simulink model "SPMSMSensorless"  (R2019b)
settings: Solver=VariableStepAuto  StartTime=0.0  StopTime=10  RelTol=1e-3
undefined symbols (not defined in the file): BmRated, DiscIntNeverNeededParam, etaFSO, etaPsiFSO, JmRated, K_dead, kFSO, KiId, KiIq, KiSpd, KpId, KpIq, kPsiFSO, KpSpd, LdRated, LqRated, OutCur_LowerLimit, OutCur_UpperLimit, OutSpd_LowerLimit, OutSpd_UpperLimit, PhiPMRated, Pn, RsRated, SetSpd_n, TsimCurLoop, TsimMotor, UdcRated, V_dead
libraries: simulink x3, eeTransforms x1, powerlib x1
(part 1 of 2)
settings Model: SimulationMode=accelerator  Creator=Downstream  LastModifiedBy=Downstream
settings DataIOCC: ReturnWorkspaceOutputs=off

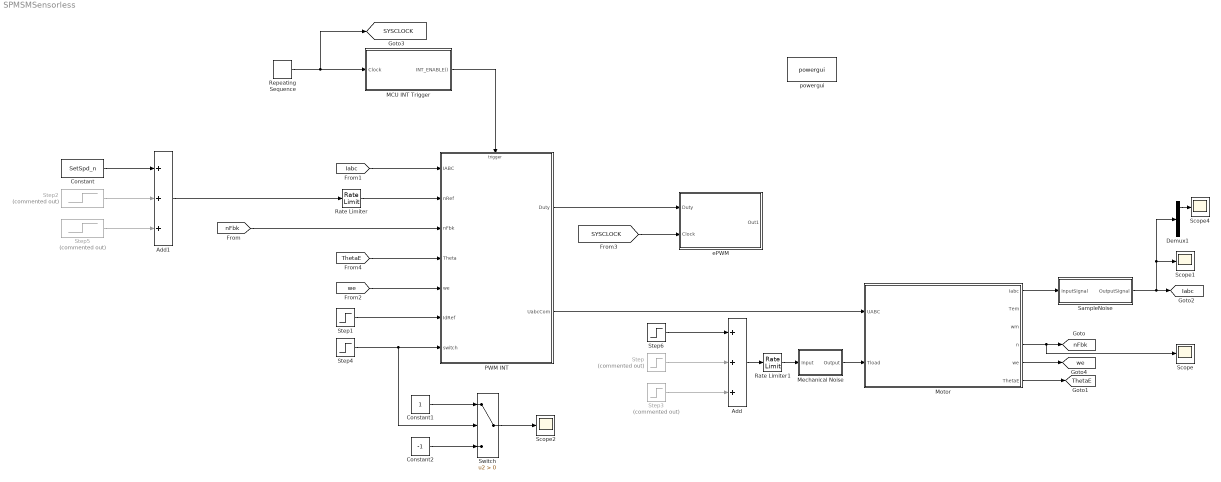
== system SPMSMSensorless ==
  Add : Sum  Inputs=+++
  Add1 : Sum  Inputs=+++
  Constant : Constant  Value=SetSpd_n  SampleTime=-1
  Constant1 : Constant
  Constant2 : Constant  Value=-1
  Demux1 : Demux  Outputs=3
  MCU INT Trigger : MATLAB Function  TreatAsAtomicUnit=on
  Mechanical Noise : Subsystem
  Motor : Subsystem
  PWM INT : Subsystem  TreatAsAtomicUnit=on
  Rate Limiter : RateLimiter  RisingSlewLimit=abs(SetSpd_n)/1  FallingSlewLimit=-abs(SetSpd_n)/1  SampleTimeMode=inherited
  Rate Limiter1 : RateLimiter  RisingSlewLimit=3  FallingSlewLimit=-3  SampleTimeMode=inherited
  Repeating Sequence : simulink/Sources/Repeating Sequence  rep_seq_t=[0 0.5*TsimCurLoop 1*TsimCurLoop]  rep_seq_y=[0 1 0]
  SampleNoise : Subsystem
  Scope{,1..2,4} (4 alike) : Scope
  Step : Step  Commented=on  Time=4  After=1.5  SampleTime=0
  Step1 : Step  Time=5  After=0  SampleTime=0
  Step2 : Step  Commented=on  Time=2  After=-SetSpd_n  SampleTime=0
  Step3 : Step  Commented=on  Time=8  After=1.5  SampleTime=0
  Step4 : Step  Time=2  Before=-1
  Step5 : Step  Commented=on  Time=6  After=-SetSpd_n  SampleTime=0
  Step6 : Step  Time=0  After=3  SampleTime=0
  Switch : Switch  Criteria=u2 > Threshold
  ePWM : Subsystem
  powergui : powerlib/powergui  Priority=1  SimulationMode=Continuous  SampleTime=50e-6  frequency=60  Iterations=50  frequencyindice=60  Pbase=100e6  ErrMax=1e-4  UnitsV=kV  UnitsW=MW  buscounter=0  FunctionMessages=off  echomessages=off  EnableUseOfTLC=off  CurrentSourceSwitches=off  DisableSnubberDevices=off  DisableRonSwitches=off  DisableVfSwitches=off  DisplayEquations=off  AutomaticDiscreteSolvers=off  SolverType=Tustin/Backward Euler (TBE)  Interpol=off  ExternalGateDelay=off  methode=off  Ts=100  x0status=blocks  SPID=on  SwTol=0  HookPort=off  NonlinearTolerance=1e-4  nMaxIteration=100  ContinueOnMaxIteration=off  RestoreLinks=warning  ResistiveCurrentMeasurement=off  Frange=[0:2:500]  Ylog=off  Xlog=on  ShowGrid=off  save=off  variable=ZData  structure=Ud_ComP  ZoomFFT=off  StartTime=2  cycles=200  DisplayStyle=3  fundamental=40  FreqAxis=on  MaxFrequency=40*4  frequencyindicesteady=1  RmsSteady=1  display=off
      settings: SourceProductName=Simscape Electrical
  tag scope: Iabc=global, SYSCLOCK=global, ThetaE=global, nFbk=global, we=global
  wires:
  MCU INT Trigger/1(INT_ENABLE()) -> PWM INT/Trigger
  Repeating Sequence/1 -> [SYSCLOCK], MCU INT Trigger/1(Clock)
  Rate Limiter/1 -> PWM INT/2(nRef)
  [ThetaE] -> PWM INT/4(Theta)
  Motor/4(n) -> Scope/1, [nFbk]
  Motor/6(ThetaE) -> [ThetaE]
  Motor/1(Iabc) -> SampleNoise/1(InputSignal)
  SampleNoise/1(OutputSignal) -> Scope1/1, Demux1/1, [Iabc]
  [Iabc] -> PWM INT/1(IABC)
  Motor/5(we) -> [we]
  [we] -> PWM INT/5(we)
  [SYSCLOCK] -> ePWM/2(Clock)
  PWM INT/1(Duty) -> ePWM/1(Duty)
  PWM INT/2(UabcCom) -> Motor/1(UABC)
  Mechanical Noise/1(Output) -> Motor/2(Tload)
  Add/1 -> Rate Limiter1/1
  Demux1/1 -> Scope4/1
  Step6/1 -> Add/1
  Step/1 -> Add/2
  Step1/1 -> PWM INT/6(IdRef)
  Add1/1 -> Rate Limiter/1
  Constant/1 -> Add1/1
  Step2/1 -> Add1/2
  Step4/1 -> Switch/2, PWM INT/7(switch)
  Constant1/1 -> Switch/1
  Constant2/1 -> Switch/3
  Switch/1 -> Scope2/1
  Step3/1 -> Add/3
  [nFbk] -> PWM INT/3(nFbk)
  Step5/1 -> Add1/3
  Rate Limiter1/1 -> Mechanical Noise/1(Input)

== system SPMSMSensorless/Mechanical Noise ==
  Input : Inport
  Add : Sum
  Gain : Gain  Gain=0.25
  Random Number : RandomNumber  Seed=1
  Rate Transition : RateTransition  OutPortSampleTime=TsimSpdLoop
  Output : Outport
  wires:
  Add/1 -> Output/1
  Input/1 -> Add/1
  Random Number/1 -> Gain/1
  Rate Transition/1 -> Add/2
  Gain/1 -> Rate Transition/1

== system SPMSMSensorless/Motor ==
  UABC : Inport
  Tload : Inport  Port=2
  Add : Sum  Inputs=+-
  Clark Transformation : Subsystem
  Demux : Demux  Outputs=3
  Electrical Model : Subsystem
  Inverse Park Transform : eeTransforms/Inverse Park Transform  AxisAlignment=D-axis  PowerInvariant=off
      settings: SourceProductName=Simscape Electrical
  "Mechanical Model " : Subsystem
  Mux : Mux  Inputs=3
  Park Transformation : Subsystem
  Scope{,1..2,4} (4 alike) : Scope
  VSINonlinearity : Subsystem  Commented=on
  Iabc : Outport
  Tem : Outport  Port=2
  wm : Outport  Port=3
  n : Outport  Port=4
  we : Outport  Port=5
  ThetaE : Outport  Port=6
  wires:
  Park Transformation/1(D) -> Scope/1, Electrical Model/1(Ud)
  "Mechanical Model "/4(we) -> Electrical Model/3(we), we/1
  Electrical Model/4(Phiq) -> "Mechanical Model "/4(Phiq)
  Electrical Model/3(Phid) -> "Mechanical Model "/3(Phid)
  Electrical Model/1(Id) -> Mux/1, Scope4/1, "Mechanical Model "/1(id)
  Park Transformation/2(Q) -> Scope2/1, Electrical Model/2(Uq)
  Demux/1 -> Clark Transformation/1(U)
  Electrical Model/2(Iq) -> Scope1/1, Mux/2, "Mechanical Model "/2(iq)
  Clark Transformation/2(Beta) -> Park Transformation/2(Beta)
  "Mechanical Model "/5(ThetaE) -> Inverse Park Transform/2, ThetaE/1, Park Transformation/3(theta)
  "Mechanical Model "/2(wm) -> wm/1
  Add/1 -> Demux/1
  Clark Transformation/1(Alpha) -> Park Transformation/1(Alpha)
  Mux/1 -> Inverse Park Transform/1
  Demux/2 -> Clark Transformation/2(V)
  Demux/3 -> Clark Transformation/3(W)
  VSINonlinearity/1(UError) -> Add/2
  "Mechanical Model "/1(Tem) -> Tem/1
  "Mechanical Model "/3(n) -> n/1
  Tload/1 -> "Mechanical Model "/5(Tload)
  Inverse Park Transform/1 -> VSINonlinearity/1(IABC), Iabc/1
  UABC/1 -> Add/1

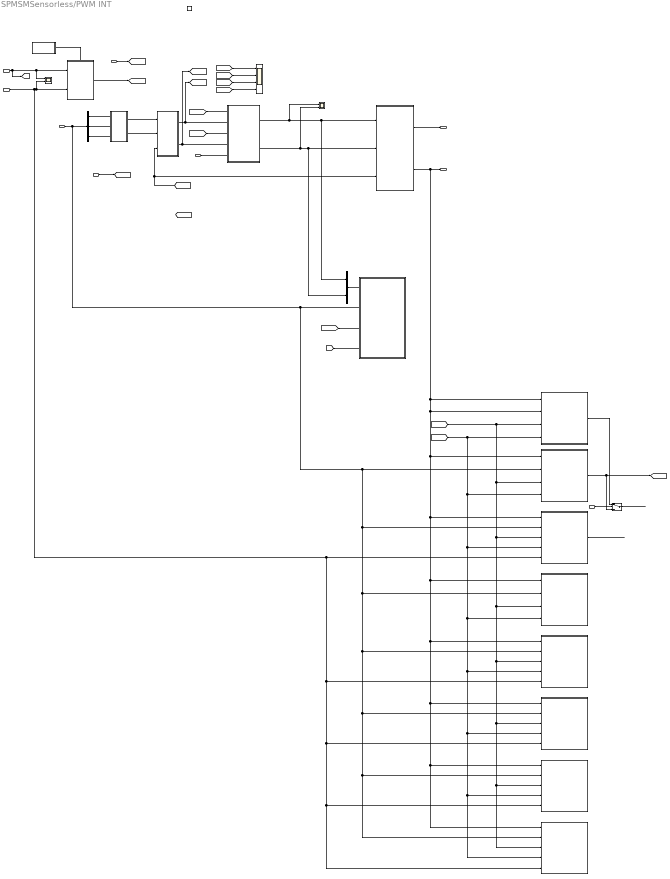
== system SPMSMSensorless/PWM INT ==
  IABC : Inport
  nRef : Inport  Port=2
  nFbk : Inport  Port=3
  Theta : Inport  Port=4
  we : Inport  Port=5
  IdRef : Inport  Port=6
  switch : Inport  Port=7
  function : TriggerPort  TriggerType=function-call  VariantControl=Variant
  Clark Transformation : Subsystem
  CurLoop : Subsystem
  Demux1 : Demux  Outputs=3
  FSO : Subsystem
  FSOLqInf : Subsystem
  FSO_Flux_SpdOb : Subsystem
  FSO_RsInf : Subsystem
  FSO_RsInfPLL : Subsystem
  MATLAB Function : MATLAB Function  TreatAsAtomicUnit=on
  Mux1 : Mux  Inputs=2
  Park Transformation : Subsystem
  PsiFSO : Subsystem
  PsiFSORsAD : Subsystem
  PsiFSORsInf : Subsystem
  "RealVoltageCompesation " : Subsystem  TreatAsAtomicUnit=on
  SVPWM : Subsystem
  Scope : Scope  NumInputPorts=4
  Scope1 : Scope  NumInputPorts=2
  Scope2 : Scope  NumInputPorts=2
  SpdLoop : Subsystem  TreatAsAtomicUnit=on
  Switch : Switch  Criteria=u2 > Threshold
  Duty : Outport
  UabcCom : Outport  Port=2
  wires:
  MATLAB Function/1(SPEED_ENABLE()) -> SpdLoop/Trigger
  nRef/1 -> [nRef], Scope1/1, SpdLoop/1(n_Ref)
  Clark Transformation/2(Beta) -> Park Transformation/2(Beta)
  Clark Transformation/1(Alpha) -> Park Transformation/1(Alpha)
  Demux1/1 -> Clark Transformation/1(U)
  Demux1/2 -> Clark Transformation/2(V)
  Demux1/3 -> Clark Transformation/3(W)
  we/1 -> CurLoop/5(we)
  Park Transformation/1(D) -> [Id_FBK], CurLoop/2(IdFbk)
  Park Transformation/2(Q) -> [Iq_FBK], CurLoop/4(IqFbk)
  SVPWM/1(Duty) -> Duty/1
  [Id_REF] -> CurLoop/1(IdRef)
  [Iq_REF] -> CurLoop/3(IqRef)
  SpdLoop/1(IqRef) -> [Iq_REF]
  IdRef/1 -> [Id_REF]
  [Iq_FBK] -> Scope/2  "IqFbk"
  [Iq_REF] -> Scope/1  "IqRef"
  Mux1/1 -> "RealVoltageCompesation "/1(Udq)
  CurLoop/2(UqCmd) -> Scope2/2, SVPWM/2(Uq), Mux1/2
  CurLoop/1(UdCmd) -> Scope2/1, SVPWM/1(Ud), Mux1/1
  [nRef] -> "RealVoltageCompesation "/4(n)
  [Theta_Est] -> "RealVoltageCompesation "/3(Theta)
  Theta/1 -> [Theta_Real]
  [Theta_Est] -> Park Transformation/3(theta), SVPWM/3(Theta)
  SVPWM/2(UabcCom) -> UabcCom/1, FSOLqInf/1(Uabc), FSOLqInf/2(Iabc), FSO/1(Uabc), PsiFSORsAD/1(Uabc), PsiFSORsInf/1(Uabc), PsiFSO/1(Uabc), FSO_RsInfPLL/1(Uabc), FSO_Flux_SpdOb/1(Uabc), FSO_RsInf/1(Uabc)
  [Id_REF] -> Scope/3  "IdRef"
  [Id_FBK] -> Scope/4  "IdFbk"
  [Theta_Real] -> PsiFSORsAD/4(ThetaReal), PsiFSORsInf/4(ThetaReal), PsiFSO/4(ThetaReal), FSO_RsInfPLL/4(ThetaReal), FSO_Flux_SpdOb/4(ThetaReal), FSO_RsInf/4(ThetaReal), FSO/4(ThetaReal), FSOLqInf/4(ThetaReal)
  [nRef] -> PsiFSO/3(nRef), PsiFSORsInf/3(nRef), PsiFSORsAD/3(nRef), FSO_RsInfPLL/3(nRef), FSO_Flux_SpdOb/3(nRef), FSO_RsInf/3(nRef), FSO/3(nRef), FSOLqInf/3(nRef)
  switch/1 -> Switch/2
  nFbk/1 -> PsiFSORsAD/5("nFbk "), PsiFSORsInf/5("nFbk "), PsiFSO/5("nFbk "), FSO_RsInfPLL/5("nFbk "), FSO_RsInf/5("nFbk "), Scope1/2, SpdLoop/2(n_Fbk)
  IABC/1 -> "RealVoltageCompesation "/2(Iuvw), FSO/2(Iabc), PsiFSORsAD/2(Iabc), PsiFSORsInf/2(Iabc), PsiFSO/2(Iabc), FSO_RsInfPLL/2(Iabc), FSO_Flux_SpdOb/2(Iabc), FSO_RsInf/2(Iabc), Demux1/1
  FSO/1(ThetaEst) -> [Theta_Est], Switch/3
  FSOLqInf/1(ThetaEst) -> Switch/1
  Switch/1 -> ?
  FSO_RsInf/1(ThetaEst) -> ?

== system SPMSMSensorless/SampleNoise ==
  InputSignal : Inport
  Add : Sum
  Add1 : Sum
  Add2 : Sum
  Demux : Demux  Outputs=3
  Gain : Gain  Gain=0.025
  Gain1 : Gain  Gain=0.025
  Gain2 : Gain  Gain=0.025
  Mux : Mux  Inputs=3
  Random Number : RandomNumber  Seed=5
  Random Number1 : RandomNumber  Seed=8
  Random Number2 : RandomNumber  Seed=15
  Scope : Scope
  OutputSignal : Outport
  wires:
  InputSignal/1 -> Demux/1
  Random Number/1 -> Gain/1
  Random Number1/1 -> Gain1/1
  Random Number2/1 -> Gain2/1
  Demux/1 -> Add/1
  Gain/1 -> Scope/1, Add/2
  Demux/2 -> Add1/1
  Demux/3 -> Add2/1
  Gain1/1 -> Add1/2
  Gain2/1 -> Add2/2
  Add/1 -> Mux/1
  Add1/1 -> Mux/2
  Add2/1 -> Mux/3
  Mux/1 -> OutputSignal/1

== system SPMSMSensorless/ePWM ==
  Duty : Inport
  Clock : Inport  Port=2
  Add : Sum  Inputs=+-
  Add1 : Sum  Inputs=+-
  Add2 : Sum  Inputs=+-
  Demux : Demux  Outputs=3
  Gain : Gain  Gain=UdcRated/2
  Mux : Mux  Inputs=3
  Relay : Relay  OnSwitchValue=0  OffSwitchValue=0  OffOutputValue=-1
  Relay1 : Relay  OnSwitchValue=0  OffSwitchValue=0  OffOutputValue=-1
  Relay2 : Relay  OnSwitchValue=0  OffSwitchValue=0  OffOutputValue=-1
  Out1 : Outport
  wires:
  Duty/1 -> Demux/1
  Demux/1 -> Add/1
  Demux/2 -> Add1/1
  Demux/3 -> Add2/1
  Clock/1 -> Add/2, Add1/2, Add2/2
  Add/1 -> Relay/1
  Add1/1 -> Relay1/1
  Add2/1 -> Relay2/1
  Relay/1 -> Mux/1
  Relay1/1 -> Mux/2
  Relay2/1 -> Mux/3
  Mux/1 -> Gain/1
  Gain/1 -> Out1/1

== system SPMSMSensorless/Motor/Clark Transformation ==
  U : Inport
  V : Inport  Port=2
  W : Inport  Port=3
  Add : Sum  Inputs=+--
  Add1 : Sum  Inputs=+-
  Gain : Gain  Gain=0.5
  Gain1 : Gain  Gain=0.5
  Gain2 : Gain  Gain=2/3
  Gain3 : Gain  Gain=2/3*0.86602540
  Alpha : Outport
  Beta : Outport  Port=2
  wires:
  V/1 -> Add1/1, Gain/1
  Gain/1 -> Add/2
  W/1 -> Add1/2, Gain1/1
  Gain1/1 -> Add/3
  U/1 -> Add/1
  Add/1 -> Gain2/1
  Gain2/1 -> Alpha/1
  Add1/1 -> Gain3/1
  Gain3/1 -> Beta/1

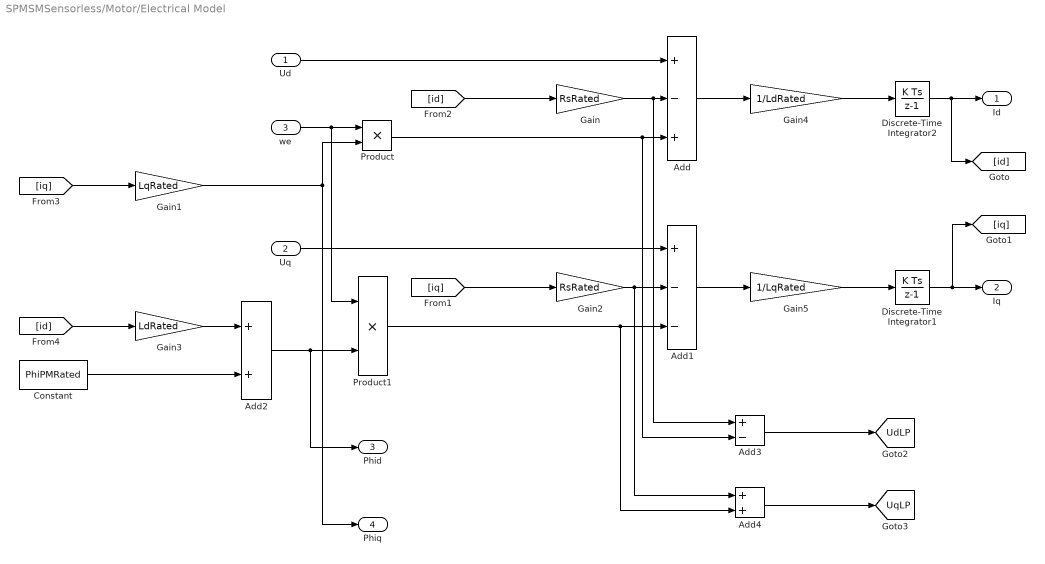
== system SPMSMSensorless/Motor/Electrical Model ==
  Ud : Inport
  Uq : Inport  Port=2
  we : Inport  Port=3
  Add : Sum  Inputs=+-+
  Add1 : Sum  Inputs=+--
  Add2 : Sum
  Add3 : Sum  Inputs=+-
  Add4 : Sum
  Constant : Constant  Value=PhiPMRated  SampleTime=TsimMotor
  Discrete-Time Integrator1 : DiscreteIntegrator  InitialCondition=1  SampleTime=TsimMotor  UpperSaturationLimit=0  LowerSaturationLimit=-400  ICPrevOutput=DiscIntNeverNeededParam  ICPrevScaledInput=DiscIntNeverNeededParam
  Discrete-Time Integrator2 : DiscreteIntegrator  InitialCondition=1  SampleTime=TsimMotor  UpperSaturationLimit=0  LowerSaturationLimit=-400  ICPrevOutput=DiscIntNeverNeededParam  ICPrevScaledInput=DiscIntNeverNeededParam
  Gain : Gain  Gain=RsRated
  Gain1 : Gain  Gain=LqRated
  Gain2 : Gain  Gain=RsRated
  Gain3 : Gain  Gain=LdRated
  Gain4 : Gain  Gain=1/LdRated
  Gain5 : Gain  Gain=1/LqRated
  Product : Product
  Product1 : Product
  Id : Outport
  Iq : Outport  Port=2
  Phid : Outport  Port=3
  Phiq : Outport  Port=4
  tag scope: UdLP=global, UqLP=global
  wires:
  Ud/1 -> Add/1
  we/1 -> Product/1, Product1/1
  Gain/1 -> Add3/1, Add/2
  [iq] -> Gain1/1
  [id] -> Gain/1
  Add/1 -> Gain4/1
  [id] -> Gain3/1
  [iq] -> Gain2/1
  Gain2/1 -> Add4/1, Add1/2
  Uq/1 -> Add1/1
  Gain3/1 -> Add2/1
  Constant/1 -> Add2/2
  Add2/1 -> Phid/1, Product1/2
  Product1/1 -> Add4/2, Add1/3
  Add1/1 -> Gain5/1
  Gain4/1 -> Discrete-Time Integrator2/1
  Gain5/1 -> Discrete-Time Integrator1/1
  Discrete-Time Integrator2/1 -> [id], Id/1
  Discrete-Time Integrator1/1 -> [iq], Iq/1
  Gain1/1 -> Phiq/1, Product/2
  Product/1 -> Add/3, Add3/2
  Add3/1 -> [UdLP]
  Add4/1 -> [UqLP]

== system SPMSMSensorless/Motor/Mechanical Model  ==
  id : Inport
  iq : Inport  Port=2
  Phid : Inport  Port=3
  Phiq : Inport  Port=4
  Tload : Inport  Port=5
  Add : Sum  Inputs=+-
  Add1 : Sum  Inputs=+--
  Discrete-Time Integrator1 : DiscreteIntegrator  SampleTime=TsimMotor  ICPrevOutput=DiscIntNeverNeededParam  ICPrevScaledInput=DiscIntNeverNeededParam
  Discrete-Time Integrator2 : DiscreteIntegrator  InitialCondition=SetSpd_n/60*2*pi  SampleTime=TsimMotor  ICPrevOutput=DiscIntNeverNeededParam  ICPrevScaledInput=DiscIntNeverNeededParam
  Gain : Gain  Gain=1.5*Pn
  Gain1 : Gain  Gain=60/2/pi
  Gain2 : Gain  Gain=Pn
  Gain3 : Gain  Gain=1/JmRated
  Gain4 : Gain  Gain=BmRated
  Product : Product
  Product1 : Product
  Tem : Outport
  wm : Outport  Port=2
  n : Outport  Port=3
  we : Outport  Port=4
  ThetaE : Outport  Port=5
  wires:
  iq/1 -> Product/1
  Phid/1 -> Product/2
  Phiq/1 -> Product1/2
  id/1 -> Product1/1
  Product/1 -> Add/1
  Product1/1 -> Add/2
  Add/1 -> Gain/1
  Gain/1 -> Tem/1, Add1/1
  Tload/1 -> Add1/2
  Add1/1 -> Gain3/1
  Gain3/1 -> Discrete-Time Integrator2/1
  Gain1/1 -> n/1
  Gain2/1 -> Discrete-Time Integrator1/1, we/1
  Discrete-Time Integrator1/1 -> ThetaE/1
  Gain4/1 -> Add1/3
  Discrete-Time Integrator2/1 -> wm/1, Gain4/1, Gain2/1, Gain1/1

== system SPMSMSensorless/Motor/Park Transformation ==
  Alpha : Inport
  Beta : Inport  Port=2
  theta : Inport  Port=3
  Add : Sum
  Add1 : Sum  Inputs=+-
  Product{,1..3} (4 alike) : Product
  Sin : Trigonometry  OutputSignalType=real
  Sin1 : Trigonometry  Operator=cos  OutputSignalType=real
  D : Outport
  Q : Outport  Port=2
  wires:
  Product/1 -> Add/1
  Sin/1 -> Product3/2, Product1/2
  Product1/1 -> Add/2
  Add1/1 -> Q/1
  Sin1/1 -> Product2/2, Product/2
  Product2/1 -> Add1/1
  Alpha/1 -> Product3/1, Product/1
  Beta/1 -> Product2/1, Product1/1
  Product3/1 -> Add1/2
  Add/1 -> D/1
  theta/1 -> Sin/1, Sin1/1

== system SPMSMSensorless/Motor/VSINonlinearity ==
  IABC : Inport
  Constant : Constant  Value=K_dead  SampleTime=TsimMotor
  Constant1 : Constant  Value=V_dead  SampleTime=TsimMotor
  Demux1 : Demux  Outputs=3
  MATLAB Function1 : MATLAB Function  TreatAsAtomicUnit=on
  MATLAB Function2 : MATLAB Function  TreatAsAtomicUnit=on
  MATLAB Function3 : MATLAB Function  TreatAsAtomicUnit=on
  Mux1 : Mux  Inputs=3
  Scope : Scope
  UError : Outport
  wires:
  Demux1/3 -> MATLAB Function3/1(I)
  Constant1/1 -> MATLAB Function3/3(Vdead), MATLAB Function2/3(Vdead), MATLAB Function1/3(Vdead)
  Constant/1 -> MATLAB Function3/2(K), MATLAB Function2/2(K), MATLAB Function1/2(K)
  MATLAB Function3/1(U) -> Mux1/3
  Demux1/2 -> MATLAB Function2/1(I)
  MATLAB Function2/1(U) -> Mux1/2
  Demux1/1 -> MATLAB Function1/1(I)
  Mux1/1 -> UError/1
  IABC/1 -> Demux1/1
  MATLAB Function1/1(U) -> Scope/1, Mux1/1

== system SPMSMSensorless/PWM INT/Clark Transformation ==
  U : Inport
  V : Inport  Port=2
  W : Inport  Port=3
  Add : Sum  Inputs=+--
  Add1 : Sum  Inputs=+-
  Gain : Gain  Gain=0.5
  Gain1 : Gain  Gain=0.5
  Gain2 : Gain  Gain=2/3
  Gain3 : Gain  Gain=2/3*0.86602540
  Alpha : Outport
  Beta : Outport  Port=2
  wires:
  V/1 -> Add1/1, Gain/1
  Gain/1 -> Add/2
  W/1 -> Add1/2, Gain1/1
  Gain1/1 -> Add/3
  U/1 -> Add/1
  Add/1 -> Gain2/1
  Gain2/1 -> Alpha/1
  Add1/1 -> Gain3/1
  Gain3/1 -> Beta/1

== system SPMSMSensorless/PWM INT/CurLoop ==
  IdRef : Inport
  IdFbk : Inport  Port=2
  IqRef : Inport  Port=3
  IqFbk : Inport  Port=4
  we : Inport  Port=5
  Add : Sum
  Constant2 : Constant  Value=PhiPMRated  SampleTime=-1
  Gain : Gain  Gain=LqRated
  Gain2 : Gain  Gain=-1
  Gain3 : Gain  Gain=LdRated
  PI_Id : Subsystem
  PI_Iq : Subsystem
  Product : Product
  Product3 : Product
  Saturation : Saturate  UpperLimit=OutCur_UpperLimit  LowerLimit=OutCur_LowerLimit
  Saturation1 : Saturate  UpperLimit=OutCur_UpperLimit  LowerLimit=OutCur_LowerLimit
  Sum : Sum  Inputs=|++
  Sum1 : Sum  Inputs=++|
  UdCmd : Outport
  UqCmd : Outport  Port=2
  wires:
  Gain/1 -> Product/1
  IdFbk/1 -> Gain3/1, PI_Id/2("Id_Fbk ")
  Sum/1 -> Saturation1/1
  PI_Id/1(PI_IdOut) -> Sum/1
  Product/1 -> Gain2/1
  IdRef/1 -> PI_Id/1(Id_Ref)
  Gain2/1 -> Sum/2
  Sum1/1 -> Saturation/1
  Saturation1/1 -> UdCmd/1
  Saturation/1 -> UqCmd/1
  IqRef/1 -> PI_Iq/1(Iq_Ref)
  PI_Iq/1(PI_IqOut) -> Sum1/2
  IqFbk/1 -> Gain/1, PI_Iq/2("Iq_Fbk ")
  Add/1 -> Product3/2
  Gain3/1 -> Add/1
  Constant2/1 -> Add/2
  Product3/1 -> Sum1/1
  we/1 -> Product3/1, Product/2

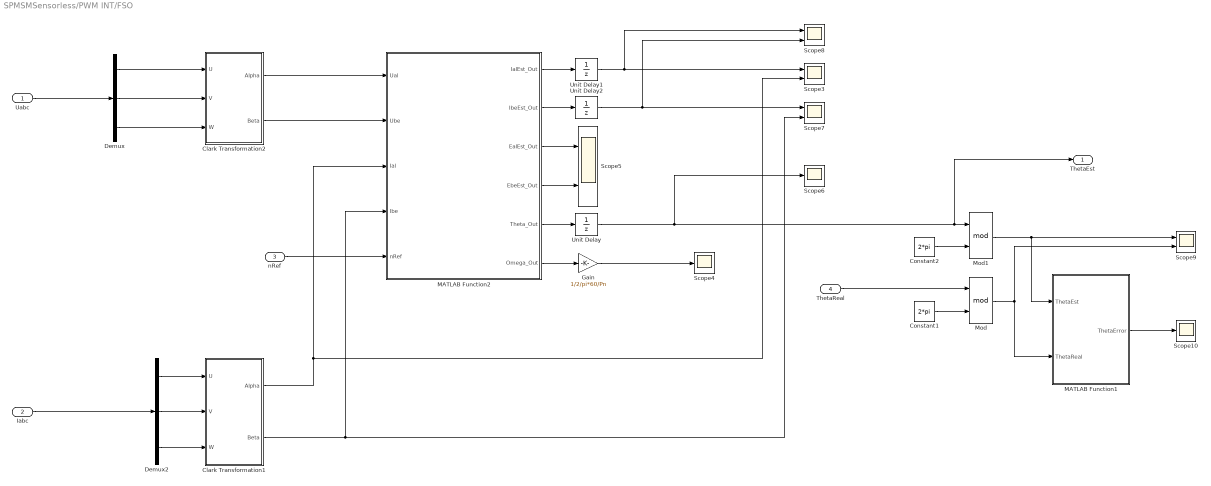
== system SPMSMSensorless/PWM INT/FSO ==
  Uabc : Inport
  Iabc : Inport  Port=2
  nRef : Inport  Port=3
  ThetaReal : Inport  Port=4
  Clark Transformation1 : Subsystem
  Clark Transformation2 : Subsystem
  Constant1 : Constant  Value=2*pi  SampleTime=-1
  Constant2 : Constant  Value=2*pi  SampleTime=-1
  Demux : Demux  Outputs=3
  Demux2 : Demux  Outputs=3
  Gain : Gain  Gain=1/2/pi*60/Pn
  MATLAB Function1 : MATLAB Function  TreatAsAtomicUnit=on
  MATLAB Function2 : MATLAB Function  TreatAsAtomicUnit=on
  Mod : Math  Operator=mod  SignedPower=off  SaturateOnIntegerOverflow=on
  Mod1 : Math  Operator=mod  SignedPower=off  SaturateOnIntegerOverflow=on
  Scope10 : Scope
  Scope{3,5,7..9} (5 alike) : Scope  NumInputPorts=2
  Scope4 : Scope
  Scope6 : Scope
  Unit Delay : UnitDelay  SampleTime=-1  HasFrameUpgradeWarning=on
  Unit Delay1 : UnitDelay  SampleTime=-1  HasFrameUpgradeWarning=on
  Unit Delay2 : UnitDelay  SampleTime=-1  HasFrameUpgradeWarning=on
  ThetaEst : Outport
  wires:
  Constant1/1 -> Mod/2
  MATLAB Function2/6(Omega_Out) -> Gain/1
  Demux2/2 -> Clark Transformation1/2(V)
  Mod1/1 -> MATLAB Function1/1(ThetaEst), Scope9/1
  Unit Delay2/1 -> Scope8/2, Scope7/1
  Clark Transformation2/2(Beta) -> MATLAB Function2/2(Ube)
  Demux2/1 -> Clark Transformation1/1(U)
  Clark Transformation1/2(Beta) -> MATLAB Function2/4(Ibe), Scope7/2
  Uabc/1 -> Demux/1
  MATLAB Function2/2(IbeEst_Out) -> Unit Delay2/1
  Iabc/1 -> Demux2/1
  MATLAB Function2/3(EalEst_Out) -> Scope5/1
  Mod/1 -> MATLAB Function1/2(ThetaReal), Scope9/2
  Demux2/3 -> Clark Transformation1/3(W)
  Demux/3 -> Clark Transformation2/3(W)
  Gain/1 -> Scope4/1
  Unit Delay1/1 -> Scope8/1, Scope3/1
  MATLAB Function2/1(IalEst_Out) -> Unit Delay1/1
  MATLAB Function1/1(ThetaError) -> Scope10/1
  Clark Transformation1/1(Alpha) -> MATLAB Function2/3(Ial), Scope3/2
  Demux/1 -> Clark Transformation2/1(U)
  MATLAB Function2/5(Theta_Out) -> Unit Delay/1
  Unit Delay/1 -> Scope6/1, ThetaEst/1, Mod1/1
  Constant2/1 -> Mod1/2
  MATLAB Function2/4(EbeEst_Out) -> Scope5/2
  Demux/2 -> Clark Transformation2/2(V)
  ThetaReal/1 -> Mod/1
  nRef/1 -> MATLAB Function2/5(nRef)
  Clark Transformation2/1(Alpha) -> MATLAB Function2/1(Ual)

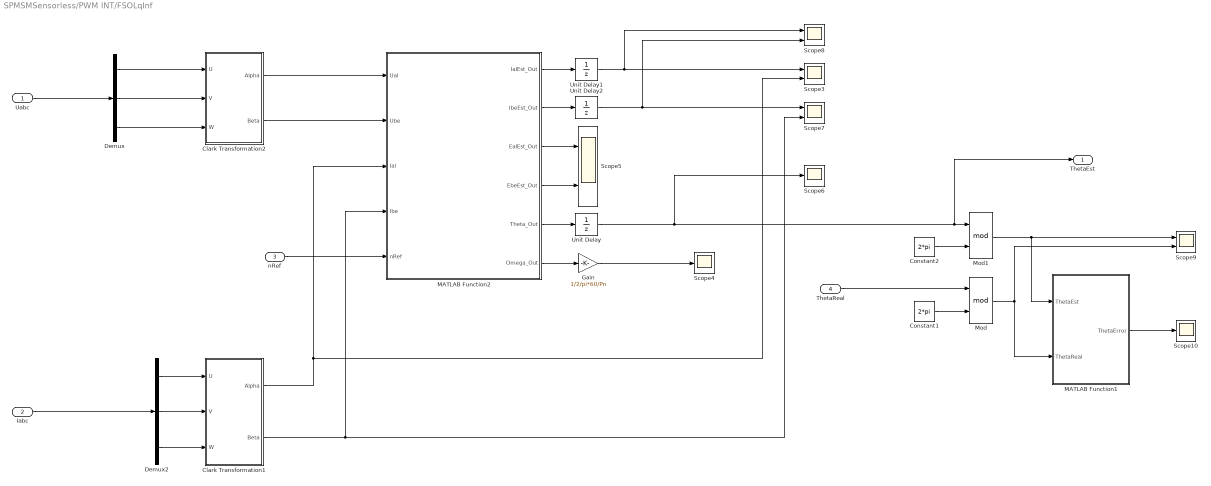
== system SPMSMSensorless/PWM INT/FSOLqInf ==
  Uabc : Inport
  Iabc : Inport  Port=2
  nRef : Inport  Port=3
  ThetaReal : Inport  Port=4
  Clark Transformation1 : Subsystem
  Clark Transformation2 : Subsystem
  Constant1 : Constant  Value=2*pi  SampleTime=-1
  Constant2 : Constant  Value=2*pi  SampleTime=-1
  Demux : Demux  Outputs=3
  Demux2 : Demux  Outputs=3
  Gain : Gain  Gain=1/2/pi*60/Pn
  MATLAB Function1 : MATLAB Function  TreatAsAtomicUnit=on
  MATLAB Function2 : MATLAB Function  TreatAsAtomicUnit=on
  Mod : Math  Operator=mod  SignedPower=off  SaturateOnIntegerOverflow=on
  Mod1 : Math  Operator=mod  SignedPower=off  SaturateOnIntegerOverflow=on
  Scope10 : Scope
  Scope{3,5,7..9} (5 alike) : Scope  NumInputPorts=2
  Scope4 : Scope
  Scope6 : Scope
  Unit Delay : UnitDelay  SampleTime=-1  HasFrameUpgradeWarning=on
  Unit Delay1 : UnitDelay  SampleTime=-1  HasFrameUpgradeWarning=on
  Unit Delay2 : UnitDelay  SampleTime=-1  HasFrameUpgradeWarning=on
  ThetaEst : Outport
  wires:
  Clark Transformation2/1(Alpha) -> MATLAB Function2/1(Ual)
  nRef/1 -> MATLAB Function2/5(nRef)
  ThetaReal/1 -> Mod/1
  Demux/2 -> Clark Transformation2/2(V)
  MATLAB Function2/4(EbeEst_Out) -> Scope5/2
  Constant2/1 -> Mod1/2
  Unit Delay/1 -> Mod1/1, ThetaEst/1, Scope6/1
  MATLAB Function2/5(Theta_Out) -> Unit Delay/1
  Demux/1 -> Clark Transformation2/1(U)
  Clark Transformation1/1(Alpha) -> Scope3/2, MATLAB Function2/3(Ial)
  MATLAB Function1/1(ThetaError) -> Scope10/1
  MATLAB Function2/1(IalEst_Out) -> Unit Delay1/1
  Unit Delay1/1 -> Scope3/1, Scope8/1
  Gain/1 -> Scope4/1
  Demux/3 -> Clark Transformation2/3(W)
  Demux2/3 -> Clark Transformation1/3(W)
  Mod/1 -> Scope9/2, MATLAB Function1/2(ThetaReal)
  MATLAB Function2/3(EalEst_Out) -> Scope5/1
  Iabc/1 -> Demux2/1
  MATLAB Function2/2(IbeEst_Out) -> Unit Delay2/1
  Uabc/1 -> Demux/1
  Clark Transformation1/2(Beta) -> Scope7/2, MATLAB Function2/4(Ibe)
  Demux2/1 -> Clark Transformation1/1(U)
  Clark Transformation2/2(Beta) -> MATLAB Function2/2(Ube)
  Unit Delay2/1 -> Scope7/1, Scope8/2
  Mod1/1 -> Scope9/1, MATLAB Function1/1(ThetaEst)
  Demux2/2 -> Clark Transformation1/2(V)
  MATLAB Function2/6(Omega_Out) -> Gain/1
  Constant1/1 -> Mod/2

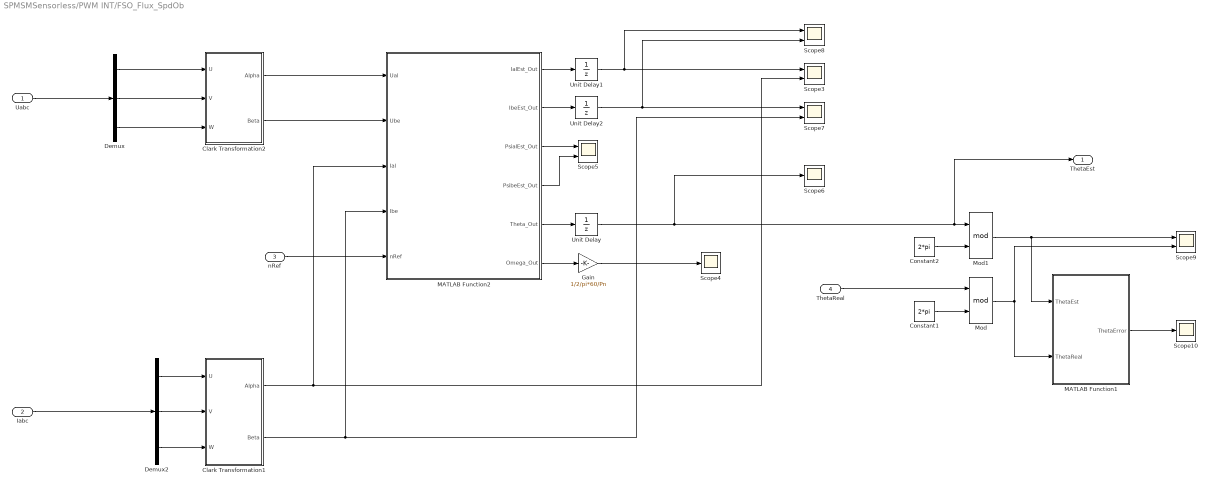
== system SPMSMSensorless/PWM INT/FSO_Flux_SpdOb ==
  Uabc : Inport
  Iabc : Inport  Port=2
  nRef : Inport  Port=3
  ThetaReal : Inport  Port=4
  Clark Transformation1 : Subsystem
  Clark Transformation2 : Subsystem
  Constant1 : Constant  Value=2*pi  SampleTime=-1
  Constant2 : Constant  Value=2*pi  SampleTime=-1
  Demux : Demux  Outputs=3
  Demux2 : Demux  Outputs=3
  Gain : Gain  Gain=1/2/pi*60/Pn
  MATLAB Function1 : MATLAB Function  TreatAsAtomicUnit=on
  MATLAB Function2 : MATLAB Function  TreatAsAtomicUnit=on
  Mod : Math  Operator=mod  SignedPower=off  SaturateOnIntegerOverflow=on
  Mod1 : Math  Operator=mod  SignedPower=off  SaturateOnIntegerOverflow=on
  Scope10 : Scope
  Scope{3,5,7..9} (5 alike) : Scope  NumInputPorts=2
  Scope4 : Scope
  Scope6 : Scope
  Unit Delay : UnitDelay  SampleTime=-1  HasFrameUpgradeWarning=on
  Unit Delay1 : UnitDelay  SampleTime=-1  HasFrameUpgradeWarning=on
  Unit Delay2 : UnitDelay  SampleTime=-1  HasFrameUpgradeWarning=on
  ThetaEst : Outport
  wires:
  Clark Transformation2/1(Alpha) -> MATLAB Function2/1(Ual)
  nRef/1 -> MATLAB Function2/5(nRef)
  ThetaReal/1 -> Mod/1
  Demux/2 -> Clark Transformation2/2(V)
  MATLAB Function2/4(PsibeEst_Out) -> Scope5/2
  Constant2/1 -> Mod1/2
  Unit Delay/1 -> Mod1/1, ThetaEst/1, Scope6/1
  MATLAB Function2/5(Theta_Out) -> Unit Delay/1
  Demux/1 -> Clark Transformation2/1(U)
  Clark Transformation1/1(Alpha) -> Scope3/2, MATLAB Function2/3(Ial)
  MATLAB Function1/1(ThetaError) -> Scope10/1
  MATLAB Function2/1(IalEst_Out) -> Unit Delay1/1
  Unit Delay1/1 -> Scope3/1, Scope8/1
  Gain/1 -> Scope4/1
  Demux/3 -> Clark Transformation2/3(W)
  Demux2/3 -> Clark Transformation1/3(W)
  Mod/1 -> Scope9/2, MATLAB Function1/2(ThetaReal)
  MATLAB Function2/3(PsialEst_Out) -> Scope5/1
  Iabc/1 -> Demux2/1
  MATLAB Function2/2(IbeEst_Out) -> Unit Delay2/1
  Uabc/1 -> Demux/1
  Clark Transformation1/2(Beta) -> Scope7/2, MATLAB Function2/4(Ibe)
  Demux2/1 -> Clark Transformation1/1(U)
  Clark Transformation2/2(Beta) -> MATLAB Function2/2(Ube)
  Unit Delay2/1 -> Scope7/1, Scope8/2
  Mod1/1 -> Scope9/1, MATLAB Function1/1(ThetaEst)
  Demux2/2 -> Clark Transformation1/2(V)
  MATLAB Function2/6(Omega_Out) -> Gain/1
  Constant1/1 -> Mod/2

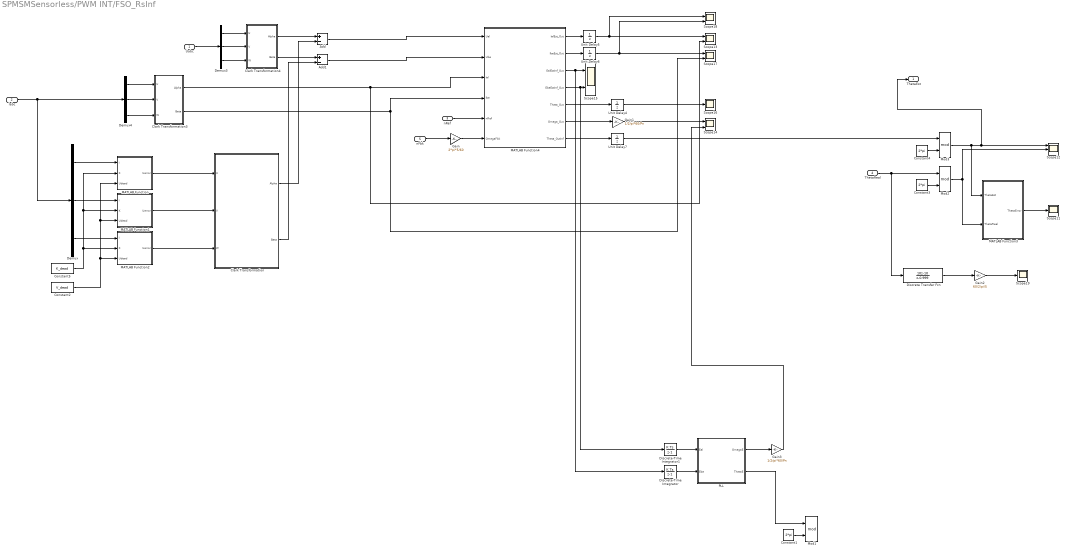
== system SPMSMSensorless/PWM INT/FSO_RsInf ==
  Uabc : Inport
  Iabc : Inport  Port=2
  nRef : Inport  Port=3
  ThetaReal : Inport  Port=4
  "nFbk " : Inport  Port=5
  Add : Sum  Inputs=+-
  Add1 : Sum  Inputs=+-
  Clark Transformation : Subsystem
  Clark Transformation3 : Subsystem
  Clark Transformation4 : Subsystem
  Constant1 : Constant  Value=2*pi  SampleTime=-1
  Constant2 : Constant  Value=V_dead  SampleTime=-1
  Constant3 : Constant  Value=2*pi  SampleTime=-1
  Constant4 : Constant  Value=2*pi  SampleTime=-1
  Constant5 : Constant  Value=K_dead  SampleTime=-1
  Demux : Demux  Outputs=3
  Demux3 : Demux  Outputs=3
  Demux4 : Demux  Outputs=3
  Discrete Transfer Fcn : DiscreteTransferFcn  Numerator=[10 -10]  Denominator=[1 -0.999]
  Discrete-Time Integrator : DiscreteIntegrator  SampleTime=-1  ICPrevOutput=DiscIntNeverNeededParam  ICPrevScaledInput=DiscIntNeverNeededParam
  Discrete-Time Integrator1 : DiscreteIntegrator  SampleTime=-1  ICPrevOutput=DiscIntNeverNeededParam  ICPrevScaledInput=DiscIntNeverNeededParam
  Gain : Gain  Gain=2*pi*5/60
  Gain1 : Gain  Gain=1/2/pi*60/Pn
  Gain2 : Gain  Gain=60/2/pi/5
  Gain3 : Gain  Gain=1/2/pi*60/Pn
  MATLAB Function : MATLAB Function  TreatAsAtomicUnit=on
  MATLAB Function1 : MATLAB Function  TreatAsAtomicUnit=on
  MATLAB Function2 : MATLAB Function  TreatAsAtomicUnit=on
  MATLAB Function3 : MATLAB Function  TreatAsAtomicUnit=on
  MATLAB Function4 : MATLAB Function  TreatAsAtomicUnit=on
  Mod1 : Math  Operator=mod  SignedPower=off  SaturateOnIntegerOverflow=on
  Mod2 : Math  Operator=mod  SignedPower=off  SaturateOnIntegerOverflow=on
  Mod3 : Math  Operator=mod  SignedPower=off  SaturateOnIntegerOverflow=on
  PLL : Subsystem
  Scope11 : Scope
  Scope12 : Scope  NumInputPorts=3
  Scope{13..15,17..18} (5 alike) : Scope  NumInputPorts=2
  Scope16 : Scope
  Scope19 : Scope
  Unit Delay{4..7} (4 alike) : UnitDelay  SampleTime=-1  HasFrameUpgradeWarning=on
  ThetaEst : Outport
  wires:
  ThetaReal/1 -> Discrete Transfer Fcn/1, Mod2/1
  Mod2/1 -> MATLAB Function3/2(ThetaReal), Scope12/2
  Demux3/2 -> Clark Transformation4/2(V)
  Constant3/1 -> Mod2/2
  Gain2/1 -> Scope19/1
  Unit Delay7/1 -> Mod3/1
  Uabc/1 -> Demux3/1
  Mod3/1 -> MATLAB Function3/1(ThetaEst), ThetaEst/1, Scope12/1
  MATLAB Function4/5(Theta_Out) -> Unit Delay4/1
  Clark Transformation3/1(Alpha) -> MATLAB Function4/3(Ial), Scope13/2
  Constant4/1 -> Mod3/2
  Unit Delay6/1 -> Scope18/2, Scope17/1
  Demux4/2 -> Clark Transformation3/2(V)
  Demux3/3 -> Clark Transformation4/3(W)
  MATLAB Function4/1(IalEst_Out) -> Unit Delay5/1
  Unit Delay4/1 -> Scope16/1
  Discrete Transfer Fcn/1 -> Gain2/1
  MATLAB Function3/1(ThetaError) -> Scope11/1
  Demux4/1 -> Clark Transformation3/1(U)
  MATLAB Function4/4(EbeEstInf_Out) -> Discrete-Time Integrator1/1, Scope15/2
  MATLAB Function4/6(Omega_Out) -> Gain1/1
  Demux3/1 -> Clark Transformation4/1(U)
  MATLAB Function4/7(Theta_OutInf) -> Unit Delay7/1
  MATLAB Function4/3(EalEstInf_Out) -> Discrete-Time Integrator/1, Scope15/1
  Demux4/3 -> Clark Transformation3/3(W)
  MATLAB Function4/2(IbeEst_Out) -> Unit Delay6/1
  Clark Transformation3/2(Beta) -> MATLAB Function4/4(Ibe), Scope17/2
  Unit Delay5/1 -> Scope13/1, Scope18/1
  Gain1/1 -> Scope14/1
  nRef/1 -> MATLAB Function4/5(nRef)
  "nFbk "/1 -> Gain/1
  Gain/1 -> MATLAB Function4/6(OmegaFbk)
  PLL/1(OmegaE) -> Gain3/1
  Gain3/1 -> Scope14/2
  Constant1/1 -> Mod1/2
  PLL/2(ThetaE) -> Mod1/1
  Discrete-Time Integrator/1 -> PLL/2(Ebe)
  Discrete-Time Integrator1/1 -> PLL/1(Eal)
  Constant2/1 -> MATLAB Function2/3(Udead), MATLAB Function1/3(Udead), MATLAB Function/3(Udead)
  Constant5/1 -> MATLAB Function2/2(K), MATLAB Function1/2(K), MATLAB Function/2(K)
  MATLAB Function2/1(Uerror) -> Clark Transformation/3(W)
  Demux/2 -> MATLAB Function1/1(I)
  Demux/1 -> MATLAB Function/1(I)
  MATLAB Function/1(Uerror) -> Clark Transformation/1(U)
  Iabc/1 -> Demux/1, Demux4/1
  MATLAB Function1/1(Uerror) -> Clark Transformation/2(V)
  Demux/3 -> MATLAB Function2/1(I)
  Clark Transformation/1(Alpha) -> Add/2
  Clark Transformation4/1(Alpha) -> Add/1
  Add/1 -> MATLAB Function4/1(Ual)
  Clark Transformation4/2(Beta) -> Add1/1
  Add1/1 -> MATLAB Function4/2(Ube)
  Clark Transformation/2(Beta) -> Add1/2

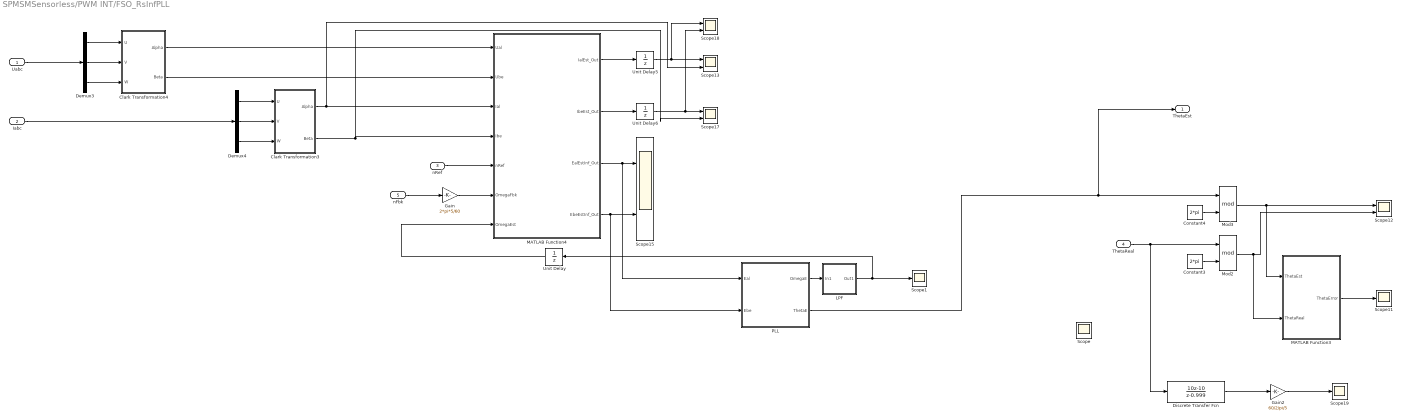
== system SPMSMSensorless/PWM INT/FSO_RsInfPLL ==
  Uabc : Inport
  Iabc : Inport  Port=2
  nRef : Inport  Port=3
  ThetaReal : Inport  Port=4
  "nFbk " : Inport  Port=5
  Clark Transformation3 : Subsystem
  Clark Transformation4 : Subsystem
  Constant3 : Constant  Value=2*pi  SampleTime=-1
  Constant4 : Constant  Value=2*pi  SampleTime=-1
  Demux3 : Demux  Outputs=3
  Demux4 : Demux  Outputs=3
  Discrete Transfer Fcn : DiscreteTransferFcn  Numerator=[10 -10]  Denominator=[1 -0.999]
  Gain : Gain  Gain=2*pi*5/60
  Gain2 : Gain  Gain=60/2/pi/5
  LPF : Subsystem
  MATLAB Function3 : MATLAB Function  TreatAsAtomicUnit=on
  MATLAB Function4 : MATLAB Function  TreatAsAtomicUnit=on
  Mod2 : Math  Operator=mod  SignedPower=off  SaturateOnIntegerOverflow=on
  Mod3 : Math  Operator=mod  SignedPower=off  SaturateOnIntegerOverflow=on
  PLL : Subsystem
  Scope{,1,11,19} (4 alike) : Scope
  Scope{12..13,15,17..18} (5 alike) : Scope  NumInputPorts=2
  Unit Delay : UnitDelay  SampleTime=-1  HasFrameUpgradeWarning=on
  Unit Delay5 : UnitDelay  SampleTime=-1  HasFrameUpgradeWarning=on
  Unit Delay6 : UnitDelay  SampleTime=-1  HasFrameUpgradeWarning=on
  ThetaEst : Outport
  wires:
  Gain/1 -> MATLAB Function4/6(OmegaFbk)
  "nFbk "/1 -> Gain/1
  Unit Delay5/1 -> Scope18/1, Scope13/1
  Clark Transformation3/2(Beta) -> Scope17/2, MATLAB Function4/4(Ibe)
  MATLAB Function4/2(IbeEst_Out) -> Unit Delay6/1
  Demux4/3 -> Clark Transformation3/3(W)
  MATLAB Function4/3(EalEstInf_Out) -> PLL/1(Eal), Scope15/1
  Demux3/1 -> Clark Transformation4/1(U)
  MATLAB Function4/4(EbeEstInf_Out) -> PLL/2(Ebe), Scope15/2
  Demux4/1 -> Clark Transformation3/1(U)
  MATLAB Function3/1(ThetaError) -> Scope11/1
  Discrete Transfer Fcn/1 -> Gain2/1
  MATLAB Function4/1(IalEst_Out) -> Unit Delay5/1
  Demux3/3 -> Clark Transformation4/3(W)
  Clark Transformation4/2(Beta) -> MATLAB Function4/2(Ube)
  Demux4/2 -> Clark Transformation3/2(V)
  Unit Delay6/1 -> Scope18/2, Scope17/1
  Constant4/1 -> Mod3/2
  Clark Transformation3/1(Alpha) -> Scope13/2, MATLAB Function4/3(Ial)
  Clark Transformation4/1(Alpha) -> MATLAB Function4/1(Ual)
  Mod3/1 -> Scope12/1, MATLAB Function3/1(ThetaEst)
  Uabc/1 -> Demux3/1
  Gain2/1 -> Scope19/1
  Constant3/1 -> Mod2/2
  Iabc/1 -> Demux4/1
  Demux3/2 -> Clark Transformation4/2(V)
  Mod2/1 -> Scope12/2, MATLAB Function3/2(ThetaReal)
  ThetaReal/1 -> Mod2/1, Discrete Transfer Fcn/1
  nRef/1 -> MATLAB Function4/5(nRef)
  PLL/2(ThetaE) -> ThetaEst/1, Mod3/1
  PLL/1(OmegaE) -> LPF/1(In1)
  Unit Delay/1 -> MATLAB Function4/7(OmegaEst)
  LPF/1(Out1) -> Unit Delay/1, Scope1/1

== system SPMSMSensorless/PWM INT/Park Transformation ==
  Alpha : Inport
  Beta : Inport  Port=2
  theta : Inport  Port=3
  Add : Sum
  Add1 : Sum  Inputs=+-
  Product{,1..3} (4 alike) : Product
  Sin : Trigonometry  OutputSignalType=real
  Sin1 : Trigonometry  Operator=cos  OutputSignalType=real
  D : Outport
  Q : Outport  Port=2
  wires:
  Product/1 -> Add/1
  Sin/1 -> Product3/2, Product1/2
  Product1/1 -> Add/2
  Add1/1 -> Q/1
  Sin1/1 -> Product2/2, Product/2
  Product2/1 -> Add1/1
  Alpha/1 -> Product3/1, Product/1
  Beta/1 -> Product2/1, Product1/1
  Product3/1 -> Add1/2
  Add/1 -> D/1
  theta/1 -> Sin/1, Sin1/1

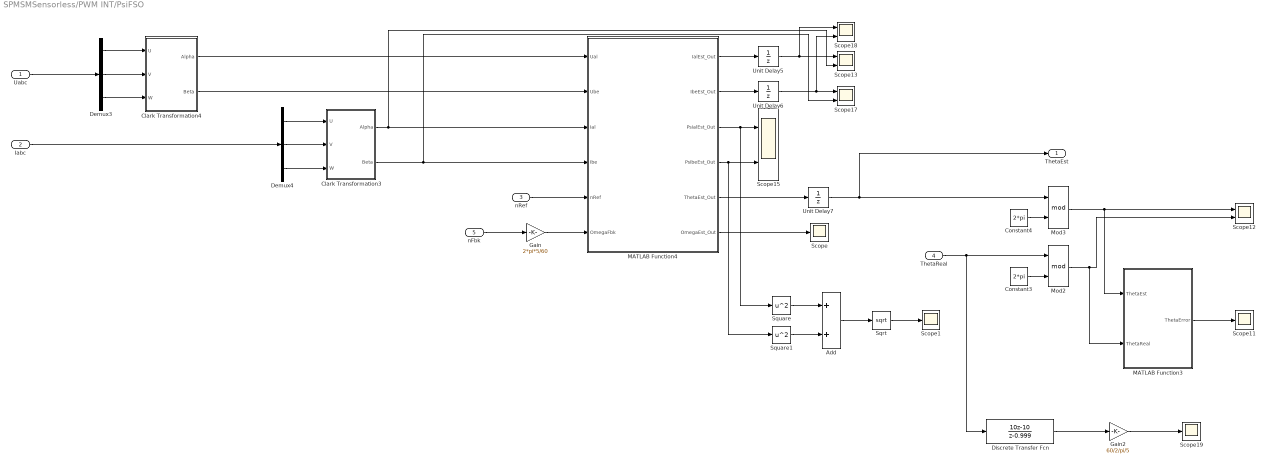
== system SPMSMSensorless/PWM INT/PsiFSO ==
  Uabc : Inport
  Iabc : Inport  Port=2
  nRef : Inport  Port=3
  ThetaReal : Inport  Port=4
  "nFbk " : Inport  Port=5
  Add : Sum
  Clark Transformation3 : Subsystem
  Clark Transformation4 : Subsystem
  Constant3 : Constant  Value=2*pi  SampleTime=-1
  Constant4 : Constant  Value=2*pi  SampleTime=-1
  Demux3 : Demux  Outputs=3
  Demux4 : Demux  Outputs=3
  Discrete Transfer Fcn : DiscreteTransferFcn  Numerator=[10 -10]  Denominator=[1 -0.999]
  Gain : Gain  Gain=2*pi*5/60
  Gain2 : Gain  Gain=60/2/pi/5
  MATLAB Function3 : MATLAB Function  TreatAsAtomicUnit=on
  MATLAB Function4 : MATLAB Function  TreatAsAtomicUnit=on
  Mod2 : Math  Operator=mod  SignedPower=off  SaturateOnIntegerOverflow=on
  Mod3 : Math  Operator=mod  SignedPower=off  SaturateOnIntegerOverflow=on
  Scope{,1,11,19} (4 alike) : Scope
  Scope{12..13,15,17..18} (5 alike) : Scope  NumInputPorts=2
  Sqrt : Sqrt  SaturateOnIntegerOverflow=on
  Square : Math  Operator=square  SignedPower=off  SaturateOnIntegerOverflow=on
  Square1 : Math  Operator=square  SignedPower=off  SaturateOnIntegerOverflow=on
  Unit Delay5 : UnitDelay  SampleTime=-1  HasFrameUpgradeWarning=on
  Unit Delay6 : UnitDelay  SampleTime=-1  HasFrameUpgradeWarning=on
  Unit Delay7 : UnitDelay  SampleTime=-1  HasFrameUpgradeWarning=on
  ThetaEst : Outport
  wires:
  nRef/1 -> MATLAB Function4/5(nRef)
  ThetaReal/1 -> Discrete Transfer Fcn/1, Mod2/1
  Mod2/1 -> MATLAB Function3/2(ThetaReal), Scope12/2
  Demux3/2 -> Clark Transformation4/2(V)
  Iabc/1 -> Demux4/1
  Constant3/1 -> Mod2/2
  Gain2/1 -> Scope19/1
  Uabc/1 -> Demux3/1
  Mod3/1 -> MATLAB Function3/1(ThetaEst), Scope12/1
  Clark Transformation4/1(Alpha) -> MATLAB Function4/1(Ual)
  Clark Transformation3/1(Alpha) -> Scope13/2, MATLAB Function4/3(Ial)
  Constant4/1 -> Mod3/2
  Unit Delay6/1 -> Scope17/1, Scope18/2
  Demux4/2 -> Clark Transformation3/2(V)
  Clark Transformation4/2(Beta) -> MATLAB Function4/2(Ube)
  Demux3/3 -> Clark Transformation4/3(W)
  MATLAB Function4/1(IalEst_Out) -> Unit Delay5/1
  Discrete Transfer Fcn/1 -> Gain2/1
  MATLAB Function3/1(ThetaError) -> Scope11/1
  Demux4/1 -> Clark Transformation3/1(U)
  MATLAB Function4/4(PsibeEst_Out) -> Square1/1, Scope15/2
  Demux3/1 -> Clark Transformation4/1(U)
  MATLAB Function4/3(PsialEst_Out) -> Square/1, Scope15/1
  Demux4/3 -> Clark Transformation3/3(W)
  MATLAB Function4/2(IbeEst_Out) -> Unit Delay6/1
  Clark Transformation3/2(Beta) -> Scope17/2, MATLAB Function4/4(Ibe)
  Unit Delay5/1 -> Scope13/1, Scope18/1
  "nFbk "/1 -> Gain/1
  Gain/1 -> MATLAB Function4/6(OmegaFbk)
  MATLAB Function4/5(ThetaEst_Out) -> Unit Delay7/1
  MATLAB Function4/6(OmegaEst_Out) -> Scope/1
  Unit Delay7/1 -> ThetaEst/1, Mod3/1
  Square/1 -> Add/1
  Square1/1 -> Add/2
  Add/1 -> Sqrt/1
  Sqrt/1 -> Scope1/1

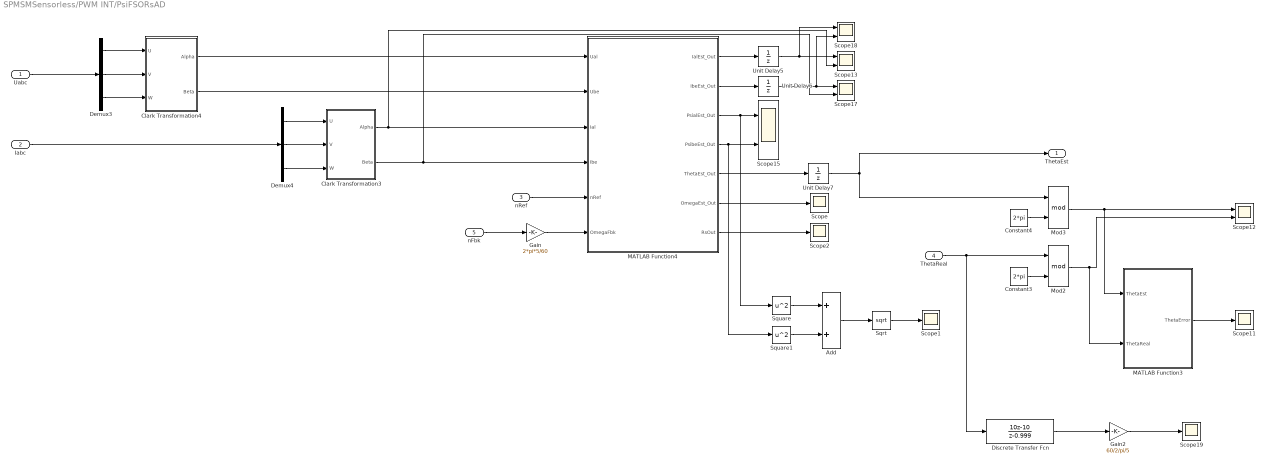
== system SPMSMSensorless/PWM INT/PsiFSORsAD ==
  Uabc : Inport
  Iabc : Inport  Port=2
  nRef : Inport  Port=3
  ThetaReal : Inport  Port=4
  "nFbk " : Inport  Port=5
  Add : Sum
  Clark Transformation3 : Subsystem
  Clark Transformation4 : Subsystem
  Constant3 : Constant  Value=2*pi  SampleTime=-1
  Constant4 : Constant  Value=2*pi  SampleTime=-1
  Demux3 : Demux  Outputs=3
  Demux4 : Demux  Outputs=3
  Discrete Transfer Fcn : DiscreteTransferFcn  Numerator=[10 -10]  Denominator=[1 -0.999]
  Gain : Gain  Gain=2*pi*5/60
  Gain2 : Gain  Gain=60/2/pi/5
  MATLAB Function3 : MATLAB Function  TreatAsAtomicUnit=on
  MATLAB Function4 : MATLAB Function  TreatAsAtomicUnit=on
  Mod2 : Math  Operator=mod  SignedPower=off  SaturateOnIntegerOverflow=on
  Mod3 : Math  Operator=mod  SignedPower=off  SaturateOnIntegerOverflow=on
  Scope{,1..2,11,19} (5 alike) : Scope
  Scope{12..13,15,17..18} (5 alike) : Scope  NumInputPorts=2
  Sqrt : Sqrt  SaturateOnIntegerOverflow=on
  Square : Math  Operator=square  SignedPower=off  SaturateOnIntegerOverflow=on
  Square1 : Math  Operator=square  SignedPower=off  SaturateOnIntegerOverflow=on
  Unit Delay5 : UnitDelay  SampleTime=-1  HasFrameUpgradeWarning=on
  Unit Delay6 : UnitDelay  SampleTime=-1  HasFrameUpgradeWarning=on
  Unit Delay7 : UnitDelay  SampleTime=-1  HasFrameUpgradeWarning=on
  ThetaEst : Outport
  wires:
  Sqrt/1 -> Scope1/1
  Add/1 -> Sqrt/1
  Square1/1 -> Add/2
  Square/1 -> Add/1
  Unit Delay7/1 -> Mod3/1, ThetaEst/1
  MATLAB Function4/6(OmegaEst_Out) -> Scope/1
  MATLAB Function4/5(ThetaEst_Out) -> Unit Delay7/1
  Gain/1 -> MATLAB Function4/6(OmegaFbk)
  "nFbk "/1 -> Gain/1
  Unit Delay5/1 -> Scope18/1, Scope13/1
  Clark Transformation3/2(Beta) -> MATLAB Function4/4(Ibe), Scope17/2
  MATLAB Function4/2(IbeEst_Out) -> Unit Delay6/1
  Demux4/3 -> Clark Transformation3/3(W)
  MATLAB Function4/3(PsialEst_Out) -> Square/1, Scope15/1
  Demux3/1 -> Clark Transformation4/1(U)
  MATLAB Function4/4(PsibeEst_Out) -> Square1/1, Scope15/2
  Demux4/1 -> Clark Transformation3/1(U)
  MATLAB Function3/1(ThetaError) -> Scope11/1
  Discrete Transfer Fcn/1 -> Gain2/1
  MATLAB Function4/1(IalEst_Out) -> Unit Delay5/1
  Demux3/3 -> Clark Transformation4/3(W)
  Clark Transformation4/2(Beta) -> MATLAB Function4/2(Ube)
  Demux4/2 -> Clark Transformation3/2(V)
  Unit Delay6/1 -> Scope18/2, Scope17/1
  Constant4/1 -> Mod3/2
  Clark Transformation3/1(Alpha) -> MATLAB Function4/3(Ial), Scope13/2
  Clark Transformation4/1(Alpha) -> MATLAB Function4/1(Ual)
  Mod3/1 -> Scope12/1, MATLAB Function3/1(ThetaEst)
  Uabc/1 -> Demux3/1
  Gain2/1 -> Scope19/1
  Constant3/1 -> Mod2/2
  Iabc/1 -> Demux4/1
  Demux3/2 -> Clark Transformation4/2(V)
  Mod2/1 -> Scope12/2, MATLAB Function3/2(ThetaReal)
  ThetaReal/1 -> Mod2/1, Discrete Transfer Fcn/1
  nRef/1 -> MATLAB Function4/5(nRef)
  MATLAB Function4/7(RsOut) -> Scope2/1

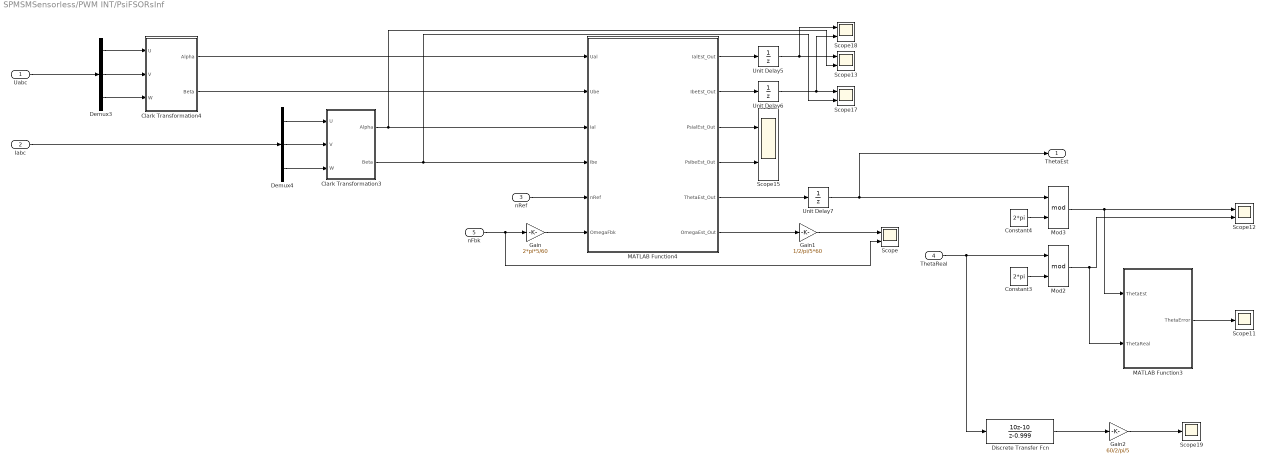
== system SPMSMSensorless/PWM INT/PsiFSORsInf ==
  Uabc : Inport
  Iabc : Inport  Port=2
  nRef : Inport  Port=3
  ThetaReal : Inport  Port=4
  "nFbk " : Inport  Port=5
  Clark Transformation3 : Subsystem
  Clark Transformation4 : Subsystem
  Constant3 : Constant  Value=2*pi  SampleTime=-1
  Constant4 : Constant  Value=2*pi  SampleTime=-1
  Demux3 : Demux  Outputs=3
  Demux4 : Demux  Outputs=3
  Discrete Transfer Fcn : DiscreteTransferFcn  Numerator=[10 -10]  Denominator=[1 -0.999]
  Gain : Gain  Gain=2*pi*5/60
  Gain1 : Gain  Gain=1/2/pi/5*60
  Gain2 : Gain  Gain=60/2/pi/5
  MATLAB Function3 : MATLAB Function  TreatAsAtomicUnit=on
  MATLAB Function4 : MATLAB Function  TreatAsAtomicUnit=on
  Mod2 : Math  Operator=mod  SignedPower=off  SaturateOnIntegerOverflow=on
  Mod3 : Math  Operator=mod  SignedPower=off  SaturateOnIntegerOverflow=on
  Scope{,12..13,15,17..18} (6 alike) : Scope  NumInputPorts=2
  Scope11 : Scope
  Scope19 : Scope
  Unit Delay5 : UnitDelay  SampleTime=-1  HasFrameUpgradeWarning=on
  Unit Delay6 : UnitDelay  SampleTime=-1  HasFrameUpgradeWarning=on
  Unit Delay7 : UnitDelay  SampleTime=-1  HasFrameUpgradeWarning=on
  ThetaEst : Outport
  wires:
  Unit Delay7/1 -> Mod3/1, ThetaEst/1
  MATLAB Function4/6(OmegaEst_Out) -> Gain1/1
  MATLAB Function4/5(ThetaEst_Out) -> Unit Delay7/1
  Gain/1 -> MATLAB Function4/6(OmegaFbk)
  "nFbk "/1 -> Scope/2, Gain/1
  Unit Delay5/1 -> Scope18/1, Scope13/1
  Clark Transformation3/2(Beta) -> MATLAB Function4/4(Ibe), Scope17/2
  MATLAB Function4/2(IbeEst_Out) -> Unit Delay6/1
  Demux4/3 -> Clark Transformation3/3(W)
  MATLAB Function4/3(PsialEst_Out) -> Scope15/1
  Demux3/1 -> Clark Transformation4/1(U)
  MATLAB Function4/4(PsibeEst_Out) -> Scope15/2
  Demux4/1 -> Clark Transformation3/1(U)
  MATLAB Function3/1(ThetaError) -> Scope11/1
  Discrete Transfer Fcn/1 -> Gain2/1
  MATLAB Function4/1(IalEst_Out) -> Unit Delay5/1
  Demux3/3 -> Clark Transformation4/3(W)
  Clark Transformation4/2(Beta) -> MATLAB Function4/2(Ube)
  Demux4/2 -> Clark Transformation3/2(V)
  Unit Delay6/1 -> Scope18/2, Scope17/1
  Constant4/1 -> Mod3/2
  Clark Transformation3/1(Alpha) -> MATLAB Function4/3(Ial), Scope13/2
  Clark Transformation4/1(Alpha) -> MATLAB Function4/1(Ual)
  Mod3/1 -> Scope12/1, MATLAB Function3/1(ThetaEst)
  Uabc/1 -> Demux3/1
  Gain2/1 -> Scope19/1
  Constant3/1 -> Mod2/2
  Iabc/1 -> Demux4/1
  Demux3/2 -> Clark Transformation4/2(V)
  Mod2/1 -> Scope12/2, MATLAB Function3/2(ThetaReal)
  ThetaReal/1 -> Mod2/1, Discrete Transfer Fcn/1
  nRef/1 -> MATLAB Function4/5(nRef)
  Gain1/1 -> Scope/1

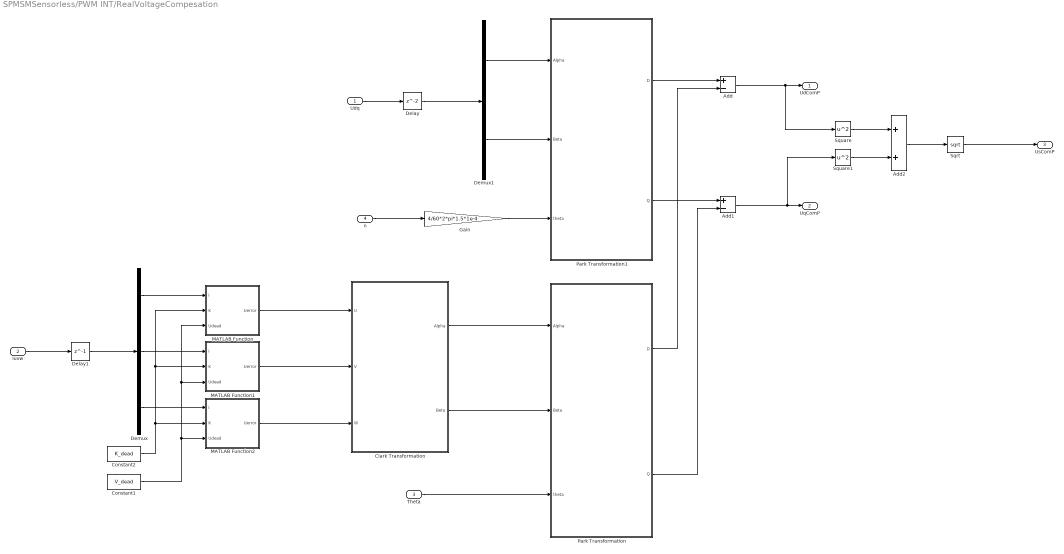
== system SPMSMSensorless/PWM INT/RealVoltageCompesation  ==
  Udq : Inport
  Iuvw : Inport  Port=2
  Theta : Inport  Port=3
  n : Inport  Port=4
  Add : Sum  Inputs=+-
  Add1 : Sum  Inputs=+-
  Add2 : Sum  AccumDataTypeStr=single  OutDataTypeStr=single
  Clark Transformation : Subsystem
  Constant1 : Constant  Value=V_dead  SampleTime=-1
  Constant2 : Constant  Value=K_dead  SampleTime=-1
  Delay : Delay
  Delay1 : Delay  DelayLength=1
  Demux : Demux  Outputs=3
  Demux1 : Demux  Outputs=2
  Gain : Gain  Gain=4/60*2*pi*1.5*1e-4
  MATLAB Function : MATLAB Function  TreatAsAtomicUnit=on
  MATLAB Function1 : MATLAB Function  TreatAsAtomicUnit=on
  MATLAB Function2 : MATLAB Function  TreatAsAtomicUnit=on
  Park Transformation : Subsystem
  Park Transformation1 : Subsystem
  Sqrt : Sqrt  OutputSignalType=real  OutDataTypeStr=single  IntermediateResultsDataTypeStr=single  SaturateOnIntegerOverflow=on
  Square : Math  Operator=square  SignedPower=off  OutputSignalType=real  OutDataTypeStr=single  SaturateOnIntegerOverflow=on
  Square1 : Math  Operator=square  SignedPower=off  OutputSignalType=real  OutDataTypeStr=single  SaturateOnIntegerOverflow=on
  UdComP : Outport
  UqComP : Outport  Port=2
  UsComP : Outport  Port=3
  wires:
  Udq/1 -> Delay/1
  Iuvw/1 -> Delay1/1
  Demux/1 -> MATLAB Function/1(I)
  Demux/2 -> MATLAB Function1/1(I)
  Demux/3 -> MATLAB Function2/1(I)
  Constant2/1 -> MATLAB Function2/2(K), MATLAB Function1/2(K), MATLAB Function/2(K)
  Constant1/1 -> MATLAB Function2/3(Udead), MATLAB Function1/3(Udead), MATLAB Function/3(Udead)
  MATLAB Function/1(Uerror) -> Clark Transformation/1(U)
  MATLAB Function1/1(Uerror) -> Clark Transformation/2(V)
  MATLAB Function2/1(Uerror) -> Clark Transformation/3(W)
  Clark Transformation/1(Alpha) -> Park Transformation/1(Alpha)
  Clark Transformation/2(Beta) -> Park Transformation/2(Beta)
  Theta/1 -> Park Transformation/3(theta)
  Delay/1 -> Demux1/1
  Park Transformation/1(D) -> Add/2
  Park Transformation/2(Q) -> Add1/2
  n/1 -> Gain/1
  Demux1/1 -> Park Transformation1/1(Alpha)
  Demux1/2 -> Park Transformation1/2(Beta)
  Gain/1 -> Park Transformation1/3(theta)
  Sqrt/1 -> UsComP/1
  Square1/1 -> Add2/2
  Add/1 -> Square/1, UdComP/1
  Square/1 -> Add2/1
  Add1/1 -> Square1/1, UqComP/1
  Add2/1 -> Sqrt/1
  Park Transformation1/1(D) -> Add/1
  Park Transformation1/2(Q) -> Add1/1
  Delay1/1 -> Demux/1

== system SPMSMSensorless/PWM INT/SVPWM ==
  Ud : Inport
  Uq : Inport  Port=2
  Theta : Inport  Port=3
  Constant : Constant  Value=0.5  SampleTime=-1
  Constant1 : Constant  Value=UdcRated/sqrt(3)  SampleTime=-1
  Demux : Demux  Outputs=2
  Divide : Product  Inputs=*/
  Gain : Gain  Gain=UdcRated/2
  Gain1 : Gain  Gain=0.5
  Gain4 : Gain  Gain=0.5
  Inverse Park Transformation : Subsystem
  MATLAB Function1 : MATLAB Function  TreatAsAtomicUnit=on
  Mux : Mux  Inputs=2
  Mux1 : Mux  Inputs=3
  Mux2 : Mux  Inputs=3
  Saturation2 : Saturate  UpperLimit=370  LowerLimit=10
  Sum : Sum  Inputs=|++
  Unit Delay : UnitDelay  SampleTime=-1  HasFrameUpgradeWarning=on
  Unit Delay1 : UnitDelay  SampleTime=-1  HasFrameUpgradeWarning=on
  Unit Delay2 : UnitDelay  SampleTime=-1  HasFrameUpgradeWarning=on
  Duty : Outport
  UabcCom : Outport  Port=2
  wires:
  Inverse Park Transformation/2(Beta) -> MATLAB Function1/2(beta)
  Divide/1 -> Demux/1
  Mux/1 -> Divide/1
  Saturation2/1 -> Divide/2
  Constant1/1 -> Saturation2/1
  Unit Delay1/1 -> Mux1/2
  Inverse Park Transformation/1(Alpha) -> MATLAB Function1/1(alpha)
  Unit Delay2/1 -> Mux1/3
  Theta/1 -> Inverse Park Transformation/3(theta)
  Demux/2 -> Inverse Park Transformation/2(Q)
  Demux/1 -> Inverse Park Transformation/1(D)
  Unit Delay/1 -> Mux1/1
  Constant/1 -> Sum/2
  Gain4/1 -> Sum/1
  Mux1/1 -> Gain4/1
  Ud/1 -> Mux/1
  Uq/1 -> Mux/2
  Sum/1 -> Duty/1
  Gain/1 -> UabcCom/1
  Gain1/1 -> Gain/1
  Mux2/1 -> Gain1/1
  MATLAB Function1/1(ta) -> Mux2/1, Unit Delay/1
  MATLAB Function1/3(tc) -> Mux2/3, Unit Delay2/1
  MATLAB Function1/2(tb) -> Unit Delay1/1, Mux2/2

== system SPMSMSensorless/PWM INT/SpdLoop ==
  n_Ref : Inport
  n_Fbk : Inport  Port=2
  function : TriggerPort  TriggerType=function-call  VariantControl=Variant
  Gain1 : Gain  Gain=2*pi/60
  Gain3 : Gain  Gain=2*pi/60
  PI_Spd : Subsystem
  IqRef : Outport
  wires:
  PI_Spd/1(PI_SpdOut) -> IqRef/1
  Gain3/1 -> PI_Spd/1(wm_Ref)
  n_Ref/1 -> Gain3/1
  n_Fbk/1 -> Gain1/1
  Gain1/1 -> PI_Spd/2("wm_Fbk ")

== system SPMSMSensorless/PWM INT/CurLoop/PI_Id ==
  Id_Ref : Inport
  "Id_Fbk " : Inport  Port=2
  Add : Sum  Inputs=+-
  Add1 : Sum
  Discrete-Time Integrator : DiscreteIntegrator  InitialCondition=TsimCurLoop  SampleTime=-1  ICPrevOutput=DiscIntNeverNeededParam  ICPrevScaledInput=DiscIntNeverNeededParam
  Gain : Gain  Gain=KpId
  Gain1 : Gain  Gain=KiId
  PI_IdOut : Outport
  wires:
  Gain/1 -> Add1/1
  Add1/1 -> PI_IdOut/1
  "Id_Fbk "/1 -> Add/2
  Add/1 -> Gain/1, Discrete-Time Integrator/1
  Gain1/1 -> Add1/2
  Id_Ref/1 -> Add/1
  Discrete-Time Integrator/1 -> Gain1/1

== system SPMSMSensorless/PWM INT/CurLoop/PI_Iq ==
  Iq_Ref : Inport
  "Iq_Fbk " : Inport  Port=2
  Add : Sum  Inputs=+-
  Add1 : Sum
  Discrete-Time Integrator : DiscreteIntegrator  InitialCondition=TsimCurLoop  SampleTime=-1  ICPrevOutput=DiscIntNeverNeededParam  ICPrevScaledInput=DiscIntNeverNeededParam
  Gain : Gain  Gain=KpIq
  Gain1 : Gain  Gain=KiIq
  PI_IqOut : Outport
  wires:
  Discrete-Time Integrator/1 -> Gain1/1
  Iq_Ref/1 -> Add/1
  Gain1/1 -> Add1/2
  Add/1 -> Discrete-Time Integrator/1, Gain/1
  "Iq_Fbk "/1 -> Add/2
  Add1/1 -> PI_IqOut/1
  Gain/1 -> Add1/1

== system SPMSMSensorless/PWM INT/FSO/Clark Transformation1 ==
  U : Inport
  V : Inport  Port=2
  W : Inport  Port=3
  Add : Sum  Inputs=+--
  Add1 : Sum  Inputs=+-
  Gain : Gain  Gain=0.5
  Gain1 : Gain  Gain=0.5
  Gain2 : Gain  Gain=2/3
  Gain3 : Gain  Gain=2/3*0.86602540
  Alpha : Outport
  Beta : Outport  Port=2
  wires:
  V/1 -> Add1/1, Gain/1
  Gain/1 -> Add/2
  W/1 -> Add1/2, Gain1/1
  Gain1/1 -> Add/3
  U/1 -> Add/1
  Add/1 -> Gain2/1
  Gain2/1 -> Alpha/1
  Add1/1 -> Gain3/1
  Gain3/1 -> Beta/1

== system SPMSMSensorless/PWM INT/FSO/Clark Transformation2 ==
  U : Inport
  V : Inport  Port=2
  W : Inport  Port=3
  Add : Sum  Inputs=+--
  Add1 : Sum  Inputs=+-
  Gain : Gain  Gain=0.5
  Gain1 : Gain  Gain=0.5
  Gain2 : Gain  Gain=2/3
  Gain3 : Gain  Gain=2/3*0.86602540
  Alpha : Outport
  Beta : Outport  Port=2
  wires:
  V/1 -> Add1/1, Gain/1
  Gain/1 -> Add/2
  W/1 -> Add1/2, Gain1/1
  Gain1/1 -> Add/3
  U/1 -> Add/1
  Add/1 -> Gain2/1
  Gain2/1 -> Alpha/1
  Add1/1 -> Gain3/1
  Gain3/1 -> Beta/1

== system SPMSMSensorless/PWM INT/FSOLqInf/Clark Transformation1 ==
  U : Inport
  V : Inport  Port=2
  W : Inport  Port=3
  Add : Sum  Inputs=+--
  Add1 : Sum  Inputs=+-
  Gain : Gain  Gain=0.5
  Gain1 : Gain  Gain=0.5
  Gain2 : Gain  Gain=2/3
  Gain3 : Gain  Gain=2/3*0.86602540
  Alpha : Outport
  Beta : Outport  Port=2
  wires:
  Gain3/1 -> Beta/1
  Add1/1 -> Gain3/1
  Gain2/1 -> Alpha/1
  Add/1 -> Gain2/1
  U/1 -> Add/1
  Gain1/1 -> Add/3
  W/1 -> Gain1/1, Add1/2
  Gain/1 -> Add/2
  V/1 -> Gain/1, Add1/1

== system SPMSMSensorless/PWM INT/FSOLqInf/Clark Transformation2 ==
  U : Inport
  V : Inport  Port=2
  W : Inport  Port=3
  Add : Sum  Inputs=+--
  Add1 : Sum  Inputs=+-
  Gain : Gain  Gain=0.5
  Gain1 : Gain  Gain=0.5
  Gain2 : Gain  Gain=2/3
  Gain3 : Gain  Gain=2/3*0.86602540
  Alpha : Outport
  Beta : Outport  Port=2
  wires:
  Gain3/1 -> Beta/1
  Add1/1 -> Gain3/1
  Gain2/1 -> Alpha/1
  Add/1 -> Gain2/1
  U/1 -> Add/1
  Gain1/1 -> Add/3
  W/1 -> Gain1/1, Add1/2
  Gain/1 -> Add/2
  V/1 -> Gain/1, Add1/1

== system SPMSMSensorless/PWM INT/FSO_Flux_SpdOb/Clark Transformation1 ==
  U : Inport
  V : Inport  Port=2
  W : Inport  Port=3
  Add : Sum  Inputs=+--
  Add1 : Sum  Inputs=+-
  Gain : Gain  Gain=0.5
  Gain1 : Gain  Gain=0.5
  Gain2 : Gain  Gain=2/3
  Gain3 : Gain  Gain=2/3*0.86602540
  Alpha : Outport
  Beta : Outport  Port=2
  wires:
  Gain3/1 -> Beta/1
  Add1/1 -> Gain3/1
  Gain2/1 -> Alpha/1
  Add/1 -> Gain2/1
  U/1 -> Add/1
  Gain1/1 -> Add/3
  W/1 -> Gain1/1, Add1/2
  Gain/1 -> Add/2
  V/1 -> Gain/1, Add1/1

== system SPMSMSensorless/PWM INT/FSO_Flux_SpdOb/Clark Transformation2 ==
  U : Inport
  V : Inport  Port=2
  W : Inport  Port=3
  Add : Sum  Inputs=+--
  Add1 : Sum  Inputs=+-
  Gain : Gain  Gain=0.5
  Gain1 : Gain  Gain=0.5
  Gain2 : Gain  Gain=2/3
  Gain3 : Gain  Gain=2/3*0.86602540
  Alpha : Outport
  Beta : Outport  Port=2
  wires:
  Gain3/1 -> Beta/1
  Add1/1 -> Gain3/1
  Gain2/1 -> Alpha/1
  Add/1 -> Gain2/1
  U/1 -> Add/1
  Gain1/1 -> Add/3
  W/1 -> Gain1/1, Add1/2
  Gain/1 -> Add/2
  V/1 -> Gain/1, Add1/1

== system SPMSMSensorless/PWM INT/FSO_RsInf/Clark Transformation ==
  U : Inport
  V : Inport  Port=2
  W : Inport  Port=3
  Add : Sum  Inputs=+--
  Add1 : Sum  Inputs=+-
  Gain : Gain  Gain=0.5
  Gain1 : Gain  Gain=0.5
  Gain2 : Gain  Gain=2/3
  Gain3 : Gain  Gain=2/3*0.86602540
  Alpha : Outport
  Beta : Outport  Port=2
  wires:
  V/1 -> Add1/1, Gain/1
  Gain/1 -> Add/2
  W/1 -> Add1/2, Gain1/1
  Gain1/1 -> Add/3
  U/1 -> Add/1
  Add/1 -> Gain2/1
  Gain2/1 -> Alpha/1
  Add1/1 -> Gain3/1
  Gain3/1 -> Beta/1

== system SPMSMSensorless/PWM INT/FSO_RsInf/Clark Transformation3 ==
  U : Inport
  V : Inport  Port=2
  W : Inport  Port=3
  Add : Sum  Inputs=+--
  Add1 : Sum  Inputs=+-
  Gain : Gain  Gain=0.5
  Gain1 : Gain  Gain=0.5
  Gain2 : Gain  Gain=2/3
  Gain3 : Gain  Gain=2/3*0.86602540
  Alpha : Outport
  Beta : Outport  Port=2
  wires:
  Gain3/1 -> Beta/1
  Add1/1 -> Gain3/1
  Gain2/1 -> Alpha/1
  Add/1 -> Gain2/1
  U/1 -> Add/1
  Gain1/1 -> Add/3
  W/1 -> Gain1/1, Add1/2
  Gain/1 -> Add/2
  V/1 -> Gain/1, Add1/1
